simulink model "uz_ssi_interface_2025b"  (R2025b)
settings: Solver=FixedStepDiscrete  StartTime=0.0  StopTime=0.005  RelTol=1e-3
values from neighbouring files (symbols this model uses):
  f_ADC = 50e3    (= 50000)    [uz_ssi_interface_init.m]
  f_clock = 100e6    (= 100000000)    [uz_ssi_interface_init.m]
  t_ADC = 1/f_ADC    (= 2e-05)    [uz_ssi_interface_init.m]
  t_clock = 1/f_clock    (= 1e-08)    [uz_ssi_interface_init.m]
undefined symbols (not defined in the file or in its folder): binary_or_gray, bit_sum, delay_first_clk_on_off, PLL, ssi_clk_divider, ssi_encoder_bit_width_multi_turn, ssi_encoder_bit_width_single_turn, ssi_encoder_number_of_status_bits
libraries: hdlsllib x92, simulink x32, simulink_extras x7, spsSampleandHoldLib x1
(part 1 of 2)
settings Model: DataTypeOverride=Off  Creator=micha  LastModifiedBy=micha
settings SolverCC: AlgebraicLoopSolver=TrustRegion
settings DataIOCC: LimitDataPoints=on  SaveOutput=off  SaveTime=off
settings OptimizationCC: BlockReduction=off  ConditionallyExecuteInputs=off  DefaultParameterBehavior=Inlined  InheritOutputTypeSmallerThanSingle=on  LifeSpan=inf
settings DebuggingCC: AlgebraicLoopMsg=error  SingleTaskRateTransMsg=error  UnconnectedInputMsg=warning  UnconnectedOutputMsg=warning  UnconnectedLineMsg=warning  AllowSymbolicDim=off  StrictBusMsg=ErrorOnBusTreatedAsVector  SFUnexpectedBacktrackingDiag=warning  SFNoUnconditionalDefaultTransitionDiag=warning  SFExecutionAtInitializationDiag=none  ArithmeticOperatorsInVariantConditions=warning
settings HardwareCC: ProdBitPerPointer=32.0  ProdBitPerSizeT=32.0  ProdBitPerPtrDiffT=32.0  ProdLargestAtomicFloat=None  ProdIntDivRoundTo=Undefined  ProdEndianess=Unspecified  ProdWordSize=32.0  ProdHWDeviceType=ASIC/FPGA->ASIC/FPGA  ProdEqTarget=off
settings ModelReferenceCC: EnableRefExpFcnMdlSchedulingChecks=on
settings SFSimCC: SimUseLocalCustomCode=off  CustomCodeUndefinedFunction=UseInterfaceOnly
settings RTWCC: RTWUseLocalCustomCode=off  GPUComputeCapability=3.5  DLArmComputeVersion=19.05
settings CodeAppCC: StateflowObjectComments=on
settings GRTTargetCC: TargetLangStandard=C89/C90 (ANSI)
settings ConfigComp: CovScope=ReferencedModels  CovMetricSettings=dw  CovSaveCumulativeToWorkspaceVar=on  CovSaveSingleToWorkspaceVar=on  CovExternalEMLEnable=off  CovSFcnEnable=off

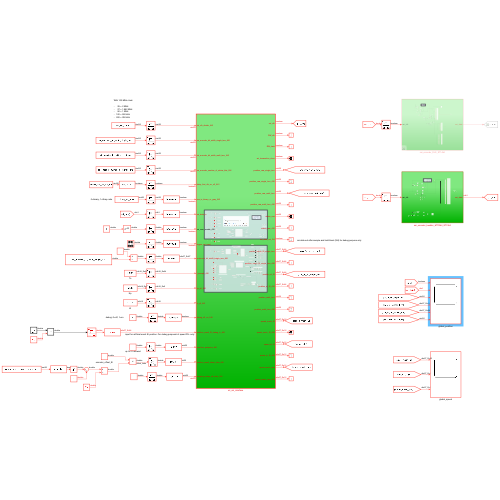
[thumbnail: Simulink's stored preview of the top-level diagram]
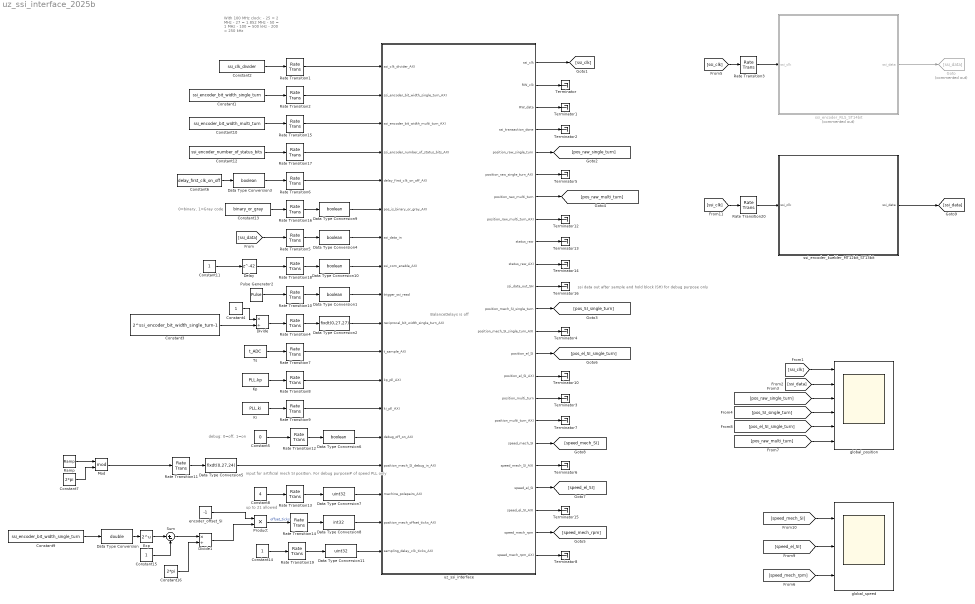
== system uz_ssi_interface_2025b ==
  note: input for artificial mech SI position. For debug purpose# of speed PLL only
  note: ssi data out after sample and hold block (SH) for debug purpose only
  note: up to 21 allowed
  note: debug: 0=off, 1=on
  note: BalanceDelays is off
  note: With 100 MHz clock:
      |
      | -     25 = 2 MHz
      | -     27 = 1.852 MHz
      | -     50 = 1 MHz
      | -   100 = 500 kHz
      | -   200 = 250 kHz
  note: 0=binary, 1=Gray code
  Constant1 : Constant  Value=ssi_encoder_bit_width_single_turn  OutDataTypeStr=uint32  SampleTime=t_clock
  Constant10 : Constant  Value=ssi_encoder_bit_width_multi_turn  OutDataTypeStr=uint32  SampleTime=t_clock
  Constant{4,11,14..15} (4 alike) : Constant  SampleTime=t_clock
  Constant12 : Constant  Value=ssi_encoder_number_of_status_bits  OutDataTypeStr=uint32  SampleTime=t_clock
  Constant13 : Constant  Value=binary_or_gray  OutDataTypeStr=uint32  SampleTime=t_clock
  Constant16 : Constant  Value=2*pi  SampleTime=t_clock
  Constant2 : Constant  Value=ssi_clk_divider  OutDataTypeStr=uint32  SampleTime=t_clock
  Constant3 : Constant  Value=2^ssi_encoder_bit_width_single_turn-1  OutDataTypeStr=double  SampleTime=t_clock
  Constant5 : Constant  Value=0  SampleTime=t_clock
  Constant6 : Constant  Value=delay_first_clk_on_off  OutDataTypeStr=uint32  SampleTime=t_clock
  Constant7 : Constant  Value=2*pi  SampleTime=t_clock
  Constant8 : Constant  Value=4  SampleTime=t_clock
  Constant9 : Constant  Value=ssi_encoder_bit_width_single_turn  OutDataTypeStr=uint32  SampleTime=t_clock
  Data Type Conversion : DataTypeConversion  OutDataTypeStr=double  SaturateOnIntegerOverflow=off  RndMeth=Floor
  Data Type Conversion{1,3..4,6,9..10} (6 alike) : DataTypeConversion  OutDataTypeStr=boolean  SaturateOnIntegerOverflow=off  RndMeth=Floor
  Data Type Conversion11 : DataTypeConversion  OutDataTypeStr=uint32  SaturateOnIntegerOverflow=off  RndMeth=Floor
  Data Type Conversion2 : DataTypeConversion  OutDataTypeStr=fixdt(0,27,27)  SaturateOnIntegerOverflow=off  RndMeth=Floor
  Data Type Conversion5 : DataTypeConversion  OutDataTypeStr=fixdt(0,27,24)  SaturateOnIntegerOverflow=off  RndMeth=Floor
  Data Type Conversion7 : DataTypeConversion  OutDataTypeStr=uint32  SaturateOnIntegerOverflow=off  RndMeth=Floor
  Data Type Conversion8 : DataTypeConversion  OutDataTypeStr=int32  SaturateOnIntegerOverflow=off  RndMeth=Floor
  Delay : Delay  DelayLength=42
  Divide : Product  Inputs=*/
  Divide1 : Product  Inputs=*/
  Exp : Math  Operator=2^u
  Goto : Goto  Commented=on  GotoTag=ssi_data
  Ki : Constant  Value=PLL.ki  OutDataTypeStr=fixdt(0,18,0)  SampleTime=-1
  Kp : Constant  Value=PLL.kp  OutDataTypeStr=fixdt(0,18,5)  SampleTime=-1
  Mod : Math  Operator=mod
  Product : Product
  Pulse Generator2 : DiscretePulseGenerator  Period=f_clock/f_ADC  PulseWidth=0.04*f_clock/f_ADC  PhaseDelay=250  SampleTime=t_clock
  Ramp : simulink/Sources/Ramp  slope=2*pi*100  start=7.5e-5  InitialOutput=0
  Rate Transition{1..20} (20 alike) : RateTransition  OutPortSampleTime=t_clock
  Sum : Sum  Inputs=|+-
  Terminator{,1..8,10,12..16} (15 alike) : Terminator
  Ts : Constant  Value=t_ADC  OutDataTypeStr=fixdt(0,18,24)  SampleTime=-1
  encoder_offset_SI : Constant  Value=-1  SampleTime=t_clock
  global_position : Scope  NumInputPorts=6
      settings: ActiveDisplayYMinimum=-0.125  ActiveDisplayYMaximum=1.125  DataLoggingVariableName=ScopeData2
  global_speed : Scope  NumInputPorts=3
      settings: ActiveDisplayYMinimum=-40.08166  ActiveDisplayYMaximum=351.59007
  ssi_encoder_RLS_ST14bit : Subsystem  Commented=on
  ssi_encoder_kuebler_MT12bit_ST13bit : Subsystem
  uz_ssi_interface : Subsystem  TreatAsAtomicUnit=on
  wires:
  Rate Transition10/1 -> Data Type Conversion1/1
  Pulse Generator2/1 -> Rate Transition10/1
  Constant2/1 -> Rate Transition1/1
  Rate Transition1/1 -> uz_ssi_interface/1(ssi_clk_divider_AXI)
  Constant1/1 -> Rate Transition2/1
  Rate Transition2/1 -> uz_ssi_interface/2(ssi_encoder_bit_width_single_turn_AXI)
  Rate Transition3/1 -> ssi_encoder_RLS_ST14bit/1(ssi_clk)
  ssi_encoder_RLS_ST14bit/1(ssi_data) -> Goto/1
  [ssi_data] -> Rate Transition5/1
  uz_ssi_interface/1(ssi_clk) -> [ssi_clk]
  uz_ssi_interface/3(RW_data) -> Terminator1/1
  uz_ssi_interface/4(ssi_transaction_done) -> Terminator2/1
  uz_ssi_interface/2(RW_clk) -> Terminator/1
  Data Type Conversion1/1 -> uz_ssi_interface/9(trigger_ssi_read)
  Rate Transition6/1 -> uz_ssi_interface/5(delay_first_clk_on_off_AXI)
  Data Type Conversion3/1 -> Rate Transition6/1
  Constant6/1 -> Data Type Conversion3/1
  uz_ssi_interface/6(position_raw_single_turn_AXI) -> Terminator5/1
  Rate Transition5/1 -> Data Type Conversion4/1
  Data Type Conversion4/1 -> uz_ssi_interface/7(ssi_data_in)
  Constant3/1 -> Divide/2
  Rate Transition4/1 -> Data Type Conversion2/1
  Data Type Conversion2/1 -> uz_ssi_interface/10(reciprocal_bit_width_single_turn_AXI)
  Constant4/1 -> Divide/1
  Divide/1 -> Rate Transition4/1
  uz_ssi_interface/13(position_mech_SI_single_turn_AXI) -> Terminator4/1
  Ts/1 -> Rate Transition7/1
  Rate Transition7/1 -> uz_ssi_interface/11(t_sample_AXI)
  Kp/1 -> Rate Transition8/1
  Rate Transition8/1 -> uz_ssi_interface/12(kp_pll_AXI)
  Ki/1 -> Rate Transition9/1
  Rate Transition9/1 -> uz_ssi_interface/13(ki_pll_AXI)
  uz_ssi_interface/18(speed_mech_SI) -> [speed_mech_SI]
  uz_ssi_interface/19(speed_mech_SI_AXI) -> Terminator6/1
  Rate Transition11/1 -> Data Type Conversion5/1
  Data Type Conversion5/1 -> uz_ssi_interface/15(position_mech_SI_debug_in_AXI)
  Data Type Conversion6/1 -> uz_ssi_interface/14(debug_off_on_AXI)
  Rate Transition12/1 -> Data Type Conversion6/1
  Constant5/1 -> Rate Transition12/1
  Mod/1 -> Rate Transition11/1
  Ramp/1 -> Mod/1
  Constant7/1 -> Mod/2
  uz_ssi_interface/23(speed_mech_rpm_AXI) -> Terminator8/1
  Rate Transition13/1 -> Data Type Conversion7/1
  Data Type Conversion7/1 -> uz_ssi_interface/16(machine_polepairs_AXI)
  Constant8/1 -> Rate Transition13/1
  Rate Transition14/1 -> Data Type Conversion8/1
  encoder_offset_SI/1 -> Product/1
  Data Type Conversion8/1 -> uz_ssi_interface/17(position_mech_offset_ticks_AXI)
  uz_ssi_interface/14(position_el_SI) -> [pos_el_SI_single_turn]
  uz_ssi_interface/15(position_el_SI_AXI) -> Terminator10/1
  Rate Transition15/1 -> uz_ssi_interface/3(ssi_encoder_bit_width_multi_turn_AXI)
  Constant10/1 -> Rate Transition15/1
  Rate Transition16/1 -> Data Type Conversion9/1
  Constant13/1 -> Rate Transition16/1
  Data Type Conversion9/1 -> uz_ssi_interface/6(pos_is_binary_or_gray_AXI)
  Rate Transition17/1 -> uz_ssi_interface/4(ssi_encoder_number_of_status_bits_AXI)
  Constant12/1 -> Rate Transition17/1
  Data Type Conversion10/1 -> uz_ssi_interface/8(ssi_com_enable_AXI)
  Rate Transition18/1 -> Data Type Conversion10/1
  Constant11/1 -> Delay/1
  uz_ssi_interface/7(position_raw_multi_turn) -> [pos_raw_multi_turn]
  uz_ssi_interface/8(position_raw_multi_turn_AXI) -> Terminator12/1
  uz_ssi_interface/9(status_raw) -> Terminator13/1
  uz_ssi_interface/10(status_raw_AXI) -> Terminator14/1
  uz_ssi_interface/21(speed_el_SI_AXI) -> Terminator15/1
  uz_ssi_interface/20(speed_el_SI) -> [speed_el_SI]
  [ssi_clk] -> global_position/1
  [ssi_data] -> global_position/2
  uz_ssi_interface/5(position_raw_single_turn) -> [pos_raw_single_turn]
  [pos_raw_single_turn] -> global_position/3
  [pos_SI_single_turn] -> global_position/4
  uz_ssi_interface/12(position_mech_SI_single_turn) -> [pos_SI_single_turn]
  uz_ssi_interface/11(ssi_data_out_SH) -> Terminator16/1
  uz_ssi_interface/22(speed_mech_rpm) -> [speed_mech_rpm]
  Delay/1 -> Rate Transition18/1
  [ssi_clk] -> Rate Transition3/1
  [speed_mech_rpm] -> global_speed/3
  [pos_raw_multi_turn] -> global_position/6
  [pos_el_SI_single_turn] -> global_position/5
  [speed_mech_SI] -> global_speed/1
  [speed_el_SI] -> global_speed/2
  Data Type Conversion11/1 -> uz_ssi_interface/18(sampling_delay_clk_ticks_AXI)
  Rate Transition19/1 -> Data Type Conversion11/1
  Constant14/1 -> Rate Transition19/1
  [ssi_clk] -> Rate Transition20/1
  Rate Transition20/1 -> ssi_encoder_kuebler_MT12bit_ST13bit/1(ssi_clk)
  ssi_encoder_kuebler_MT12bit_ST13bit/1(ssi_data) -> [ssi_data]
  uz_ssi_interface/16(position_multi_turn) -> Terminator3/1
  uz_ssi_interface/17(position_multi_turn_AXI) -> Terminator7/1
  Product/1 -> Rate Transition14/1  "offset_ticks"
  Constant9/1 -> Data Type Conversion/1
  Constant15/1 -> Sum/2
  Exp/1 -> Sum/1
  Sum/1 -> Divide1/1
  Constant16/1 -> Divide1/2
  Divide1/1 -> Product/2
  Data Type Conversion/1 -> Exp/1

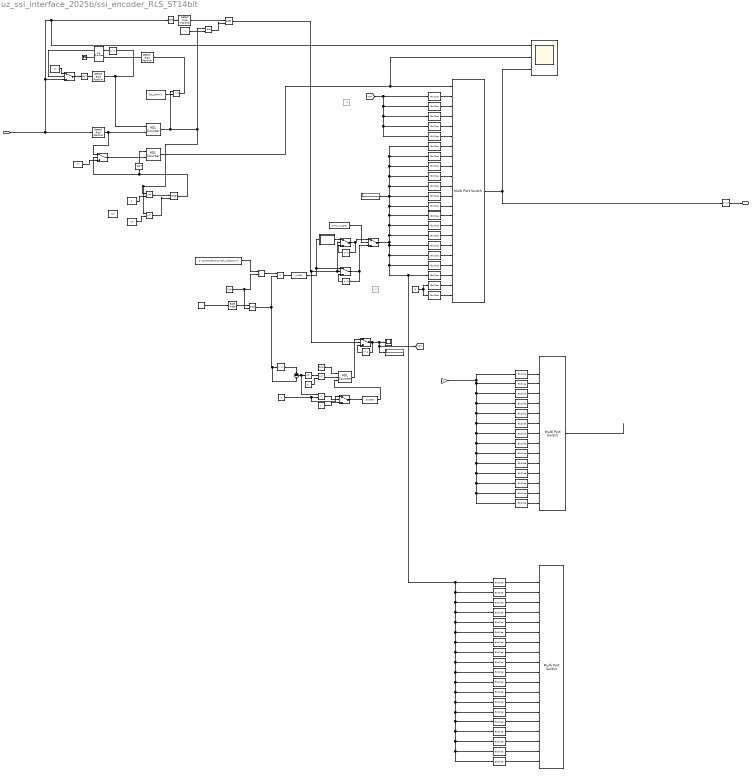
== system uz_ssi_interface_2025b/ssi_encoder_RLS_ST14bit ==
  note: 5bit multiturn, 14bit single turn 2bit status
  note: 14 bit single turn
  note: multiturn information
  note: 170 ns delay of the readhead
  note: Detect first falling edge of the clock
  note: singleturn information
  note: 19 bit single turn
  ssi_clk : Inport
  AND : Logic  IconShape=distinctive  AllPortsSameDT=off  OutDataTypeStr=boolean
  AND1 : Logic  IconShape=distinctive  AllPortsSameDT=off  OutDataTypeStr=boolean
  Abs : Abs  SaturateOnIntegerOverflow=off
  Bit Slice{1,14,19,26,40} (5 alike) : hdlsllib/Logic and Bit Operations/Bit Slice  lidx=1  ridx=1
  Bit Slice10 : hdlsllib/Logic and Bit Operations/Bit Slice  lidx=5  ridx=5
  Bit Slice{11,16,23,37} (4 alike) : hdlsllib/Logic and Bit Operations/Bit Slice  lidx=4  ridx=4
  Bit Slice{12,17,24,38} (4 alike) : hdlsllib/Logic and Bit Operations/Bit Slice  lidx=3  ridx=3
  Bit Slice{13,18,25,39} (4 alike) : hdlsllib/Logic and Bit Operations/Bit Slice  lidx=2  ridx=2
  Bit Slice{15,20..21,27,41} (5 alike) : hdlsllib/Logic and Bit Operations/Bit Slice  lidx=0  ridx=0
  Bit Slice2 : hdlsllib/Logic and Bit Operations/Bit Slice  lidx=13  ridx=13
  Bit Slice22 : hdlsllib/Logic and Bit Operations/Bit Slice  lidx=5  ridx=5
  Bit Slice28 : hdlsllib/Logic and Bit Operations/Bit Slice  lidx=13  ridx=13
  Bit Slice29 : hdlsllib/Logic and Bit Operations/Bit Slice  lidx=12  ridx=12
  Bit Slice3 : hdlsllib/Logic and Bit Operations/Bit Slice  lidx=12  ridx=12
  Bit Slice30 : hdlsllib/Logic and Bit Operations/Bit Slice  lidx=11  ridx=11
  Bit Slice31 : hdlsllib/Logic and Bit Operations/Bit Slice  lidx=10  ridx=10
  Bit Slice32 : hdlsllib/Logic and Bit Operations/Bit Slice  lidx=9  ridx=9
  Bit Slice33 : hdlsllib/Logic and Bit Operations/Bit Slice  lidx=8  ridx=8
  Bit Slice34 : hdlsllib/Logic and Bit Operations/Bit Slice  lidx=7  ridx=7
  Bit Slice35 : hdlsllib/Logic and Bit Operations/Bit Slice  lidx=6  ridx=6
  Bit Slice36 : hdlsllib/Logic and Bit Operations/Bit Slice  lidx=5  ridx=5
  Bit Slice4 : hdlsllib/Logic and Bit Operations/Bit Slice  lidx=11  ridx=11
  Bit Slice42 : hdlsllib/Logic and Bit Operations/Bit Slice  lidx=13  ridx=13
  Bit Slice43 : hdlsllib/Logic and Bit Operations/Bit Slice  lidx=12  ridx=12
  Bit Slice44 : hdlsllib/Logic and Bit Operations/Bit Slice  lidx=11  ridx=11
  Bit Slice45 : hdlsllib/Logic and Bit Operations/Bit Slice  lidx=10  ridx=10
  Bit Slice46 : hdlsllib/Logic and Bit Operations/Bit Slice  lidx=9  ridx=9
  Bit Slice47 : hdlsllib/Logic and Bit Operations/Bit Slice  lidx=8  ridx=8
  Bit Slice48 : hdlsllib/Logic and Bit Operations/Bit Slice  lidx=7  ridx=7
  Bit Slice49 : hdlsllib/Logic and Bit Operations/Bit Slice  lidx=6  ridx=6
  Bit Slice5 : hdlsllib/Logic and Bit Operations/Bit Slice  lidx=10  ridx=10
  Bit Slice50 : hdlsllib/Logic and Bit Operations/Bit Slice  lidx=18  ridx=18
  Bit Slice51 : hdlsllib/Logic and Bit Operations/Bit Slice  lidx=17  ridx=17
  Bit Slice52 : hdlsllib/Logic and Bit Operations/Bit Slice  lidx=16  ridx=16
  Bit Slice53 : hdlsllib/Logic and Bit Operations/Bit Slice  lidx=15  ridx=15
  Bit Slice54 : hdlsllib/Logic and Bit Operations/Bit Slice  lidx=14  ridx=14
  Bit Slice6 : hdlsllib/Logic and Bit Operations/Bit Slice  lidx=9  ridx=9
  Bit Slice7 : hdlsllib/Logic and Bit Operations/Bit Slice  lidx=8  ridx=8
  Bit Slice8 : hdlsllib/Logic and Bit Operations/Bit Slice  lidx=7  ridx=7
  Bit Slice9 : hdlsllib/Logic and Bit Operations/Bit Slice  lidx=6  ridx=6
  Constant : Constant  Value=bit_sum+1  SampleTime=t_clock
  Constant1 : Constant  Value=0  SampleTime=t_clock
  Constant10 : Constant  Value=false  SampleTime=t_clock
  Constant11 : Constant  Value=0  SampleTime=t_clock
  Constant12 : Constant  SampleTime=t_clock
  Constant13 : Constant  Value=0  OutDataTypeStr=uint32  SampleTime=t_clock
  Constant14 : Constant  Commented=on  Value=19  OutDataTypeStr=uint32  SampleTime=t_clock
  Constant15 : Constant  Value=binary_or_gray  SampleTime=t_clock
  Constant16 : Constant  Value=15  SampleTime=t_clock
  Constant2 : Constant  SampleTime=t_clock
  Constant3 : Constant  Value=0  OutDataTypeStr=boolean  SampleTime=t_clock
  Constant4 : Constant  Value=5  SampleTime=t_clock
  Constant5 : Constant  Value=2  SampleTime=t_clock
  Constant6 : Constant  Commented=on  Value=3875  OutDataTypeStr=uint32  SampleTime=t_clock
  Constant7 : Constant  Value=2*pi  SampleTime=t_clock
  Constant8 : Constant  Value=22  SampleTime=t_clock
  Constant9 : Constant  Value=2^ssi_encoder_bit_width_single_turn-1  SampleTime=t_clock
  Data Type Conversion : DataTypeConversion  OutDataTypeStr=uint32  SaturateOnIntegerOverflow=off  RndMeth=Floor
  Data Type Conversion1 : DataTypeConversion  OutDataTypeStr=boolean  SaturateOnIntegerOverflow=off  RndMeth=Floor
  Delay : Delay  DelayLength=1
  Delay1 : Delay  DelayLength=17  SampleTime=t_clock
  Delay2 : Delay  DelayLength=1  SampleTime=t_clock
  Delay3 : Delay  DelayLength=1
  Delay4 : Delay  DelayLength=1  InitialCondition=19  SampleTime=t_clock
  Delay5 : Delay  DelayLength=1  SampleTime=t_clock
  Detect Rise Positive{,1..3} (4 alike) : simulink/Logic and Bit Operations/Detect Rise Positive  vinit=0  OutDataTypeStr=boolean
  Display : Display
  Display1 : Display
  Divide : Product  Inputs=*/
  Gain : Gain
  HDL Counter : hdlsllib/Sources/HDL Counter  CountType=Count limited  CountInit=0  CountStep=1  CountMax=bit_sum+1  CountFromType=Initial value  CountFrom=0  CountResetPort=on  CountLoadPort=off  CountEnbPort=on  CountDirPort=off  CountHitOutputPort=off  CountDataType=Unsigned  CountWordLen=8  CountFracLen=0  CountSampTime=t_clock
  HDL Counter1 : hdlsllib/Sources/HDL Counter  CountType=Count limited  CountInit=0  CountStep=1  CountMax=bit_sum+1  CountFromType=Initial value  CountFrom=0  CountResetPort=on  CountLoadPort=off  CountEnbPort=on  CountDirPort=off  CountHitOutputPort=off  CountDataType=Unsigned  CountWordLen=8  CountFracLen=0  CountSampTime=t_clock
  HDL Counter2 : hdlsllib/Sources/HDL Counter  CountType=Count limited  CountInit=19  CountStep=1  CountMax=ssi_encoder_bit_width_multi_turn  CountFromType=Initial value  CountFrom=19  CountResetPort=on  CountLoadPort=off  CountEnbPort=on  CountDirPort=on  CountHitOutputPort=off  CountDataType=Unsigned  CountWordLen=5  CountFracLen=0  CountSampTime=t_clock
  Index Vector : MultiPortSwitch  DataPortOrder=Zero-based contiguous  Inputs=21  zeroidx=on  SaturateOnIntegerOverflow=off  InputSameDT=off
  Index Vector1 : MultiPortSwitch  DataPortOrder=Zero-based contiguous  Inputs=14  zeroidx=on  SaturateOnIntegerOverflow=off  InputSameDT=off
  Index Vector2 : MultiPortSwitch  DataPortOrder=Zero-based contiguous  Inputs=19  zeroidx=on  SaturateOnIntegerOverflow=off  InputSameDT=off
  MATLAB Function : MATLAB Function  TreatAsAtomicUnit=on
  Mod : Math  Operator=mod
  NOT : Logic  Operator=NOT  IconShape=distinctive  AllPortsSameDT=off  OutDataTypeStr=boolean
  NOT1 : Logic  Operator=NOT  IconShape=distinctive  AllPortsSameDT=off  OutDataTypeStr=boolean
  NOT2 : Logic  Operator=NOT  IconShape=distinctive  AllPortsSameDT=off  OutDataTypeStr=boolean
  Product : Product
  Ramp : simulink/Sources/Ramp  slope=-2*pi*50  start=7.5e-5  InitialOutput=0
  Rate Transition : RateTransition  OutPortSampleTime=t_clock
  Relational Operator : RelationalOperator  OutDataTypeStr=boolean  RndMeth=Simplest  InputSameDT=off
  Relational Operator1 : RelationalOperator  OutDataTypeStr=boolean  RndMeth=Simplest  InputSameDT=off
  Relational Operator2 : RelationalOperator  Operator===  OutDataTypeStr=boolean  RndMeth=Simplest  InputSameDT=off
  Relational Operator3 : RelationalOperator  Operator=<=  OutDataTypeStr=boolean  RndMeth=Simplest  InputSameDT=off
  Relational Operator4 : RelationalOperator  OutDataTypeStr=boolean  RndMeth=Simplest  InputSameDT=off
  Relational Operator5 : RelationalOperator  Operator=<  OutDataTypeStr=boolean  RndMeth=Simplest  InputSameDT=off
  S-R Flip-Flop : simulink_extras/Flip Flops/S-R Flip-Flop  initial_condition=0
  Scope : Scope  NumInputPorts=3
      settings: ActiveDisplayYMinimum=-2.5  ActiveDisplayYMaximum=22.5
  Scope1 : Scope
  Sum : Sum  Inputs=+-
  Switch{,1..6} (7 alike) : Switch  Criteria=u2 > Threshold  SaturateOnIntegerOverflow=off  InputSameDT=off
  Terminator : Terminator
  ssi_data : Outport
  wires:
  NOT/1 -> Detect Rise Positive/1
  Constant/1 -> Relational Operator/2
  Switch/1 -> NOT/1
  S-R Flip-Flop/1 -> Switch/2
  Delay/1 -> S-R Flip-Flop/1
  Relational Operator/1 -> Detect Rise Positive2/1
  Detect Rise Positive2/1 -> S-R Flip-Flop/2
  Detect Rise Positive/1 -> HDL Counter/1, Delay/1
  Relational Operator2/1 -> AND/2
  Constant2/1 -> Relational Operator2/2
  NOT1/1 -> Detect Rise Positive3/1
  Detect Rise Positive3/1 -> AND/1
  Detect Rise Positive1/1 -> HDL Counter/2, Switch3/1
  HDL Counter/1 -> Relational Operator3/1, Relational Operator1/1, Relational Operator2/1, Relational Operator/1
  S-R Flip-Flop/2 -> Terminator/1
  Constant1/1 -> Switch/1
  ssi_clk/1 -> Scope/1, NOT1/1, Switch/3, Detect Rise Positive1/1
  Relational Operator1/1 -> AND1/1
  AND1/1 -> NOT2/1, Switch3/2
  Constant5/1 -> Relational Operator1/2
  Relational Operator3/1 -> AND1/2
  Constant16/1 -> Relational Operator3/2
  Switch3/1 -> HDL Counter1/2
  NOT2/1 -> HDL Counter1/1
  Ramp/1 -> Rate Transition/1
  Constant9/1 -> Divide/1
  Divide/1 -> Product/1
  Constant7/1 -> Mod/2, Divide/2
  Product/1 -> Data Type Conversion/1
  Rate Transition/1 -> Mod/1
  Delay2/1 -> Switch1/3
  Data Type Conversion/1 -> Switch1/1, MATLAB Function/1(u)
  AND/1 -> Switch2/2, Switch6/2, Switch1/2
  Constant3/1 -> Switch3/3
  HDL Counter1/1 -> Scope/2, Index Vector/1
  Delay1/1 -> ssi_data/1
  Delay3/1 -> Sum/1
  Mod/1 -> Sum/2, Delay3/1, Product/2
  Sum/1 -> Relational Operator5/1, Abs/1
  Abs/1 -> Relational Operator4/1
  Constant4/1 -> Relational Operator4/2
  Relational Operator4/1 -> HDL Counter2/2
  HDL Counter2/1 -> Switch2/1
  Delay4/1 -> Switch2/3
  Switch2/1 -> [MT], Display1/1, Scope1/1, Delay4/1
  Constant10/1 -> HDL Counter2/1
  Constant11/1 -> Switch4/1, Relational Operator5/2
  Relational Operator5/1 -> Switch4/2
  Switch4/1 -> Data Type Conversion1/1
  Constant12/1 -> Switch4/3
  [MT] -> Bit Slice17/1, Bit Slice18/1, Bit Slice19/1, Bit Slice20/1, Bit Slice16/1
  Bit Slice16/1 -> Index Vector/2
  Bit Slice17/1 -> Index Vector/3
  Bit Slice18/1 -> Index Vector/4
  Bit Slice19/1 -> Index Vector/5
  Bit Slice20/1 -> Index Vector/6
  Bit Slice2/1 -> Index Vector/7
  Bit Slice3/1 -> Index Vector/8
  Bit Slice4/1 -> Index Vector/9
  Bit Slice5/1 -> Index Vector/10
  Bit Slice6/1 -> Index Vector/11
  Bit Slice7/1 -> Index Vector/12
  Bit Slice8/1 -> Index Vector/13
  Bit Slice9/1 -> Index Vector/14
  Bit Slice10/1 -> Index Vector/15
  Bit Slice11/1 -> Index Vector/16
  Bit Slice12/1 -> Index Vector/17
  Bit Slice13/1 -> Index Vector/18
  Bit Slice14/1 -> Index Vector/19
  Bit Slice15/1 -> Index Vector/20
  Bit Slice1/1 -> Index Vector/21
  Bit Slice21/1 -> Index Vector/22
  Constant13/1 -> Bit Slice1/1, Bit Slice21/1
  Data Type Conversion1/1 -> HDL Counter2/3
  Constant15/1 -> Switch5/2
  Switch1/1 -> Delay2/1, Switch5/3
  MATLAB Function/1(y) -> Switch6/1
  Switch6/1 -> Delay5/1, Switch5/1
  Delay5/1 -> Switch6/3
  Bit Slice29/1 -> Index Vector1/3
  Bit Slice33/1 -> Index Vector1/7
  Bit Slice26/1 -> Index Vector1/14
  Bit Slice22/1 -> Index Vector1/10
  Bit Slice28/1 -> Index Vector1/2
  Bit Slice34/1 -> Index Vector1/8
  Bit Slice23/1 -> Index Vector1/11
  Bit Slice31/1 -> Index Vector1/5
  Bit Slice27/1 -> Index Vector1/15
  Bit Slice35/1 -> Index Vector1/9
  Bit Slice30/1 -> Index Vector1/4
  Bit Slice32/1 -> Index Vector1/6
  Bit Slice25/1 -> Index Vector1/13
  Bit Slice24/1 -> Index Vector1/12
  Index Vector1/1 -> ?
  Bit Slice47/1 -> Index Vector2/12
  Bit Slice37/1 -> Index Vector2/16
  Bit Slice40/1 -> Index Vector2/19
  Bit Slice36/1 -> Index Vector2/15
  Bit Slice44/1 -> Index Vector2/9
  Bit Slice41/1 -> Index Vector2/20
  Bit Slice42/1 -> Index Vector2/7
  Bit Slice38/1 -> Index Vector2/17
  Bit Slice45/1 -> Index Vector2/10
  Bit Slice46/1 -> Index Vector2/11
  Bit Slice48/1 -> Index Vector2/13
  Bit Slice43/1 -> Index Vector2/8
  Bit Slice49/1 -> Index Vector2/14
  Bit Slice39/1 -> Index Vector2/18
  Bit Slice52/1 -> Index Vector2/4
  Bit Slice53/1 -> Index Vector2/5
  Bit Slice50/1 -> Index Vector2/2
  Bit Slice54/1 -> Index Vector2/6
  Bit Slice51/1 -> Index Vector2/3
  Switch5/1 -> Bit Slice37/1, Bit Slice38/1, Bit Slice39/1, Bit Slice40/1, Bit Slice41/1, Bit Slice36/1, Bit Slice49/1, Bit Slice48/1, Bit Slice47/1, Bit Slice46/1, Bit Slice45/1, Bit Slice44/1, Bit Slice43/1, Bit Slice42/1, Bit Slice54/1, Bit Slice53/1, Bit Slice52/1, Bit Slice51/1, Bit Slice50/1, Bit Slice15/1, Bit Slice14/1, Bit Slice13/1, Bit Slice12/1, Display/1, Bit Slice6/1, Bit Slice5/1, Bit Slice4/1, Bit Slice2/1, Bit Slice3/1, Bit Slice7/1, Bit Slice8/1, Bit Slice9/1, Bit Slice10/1, Bit Slice11/1
  Index Vector/1 -> Scope/3, Delay1/1
  Gain/1 -> Bit Slice28/1, Bit Slice27/1, Bit Slice26/1, Bit Slice25/1, Bit Slice24/1, Bit Slice23/1, Bit Slice22/1, Bit Slice35/1, Bit Slice34/1, Bit Slice33/1, Bit Slice32/1, Bit Slice31/1, Bit Slice30/1, Bit Slice29/1

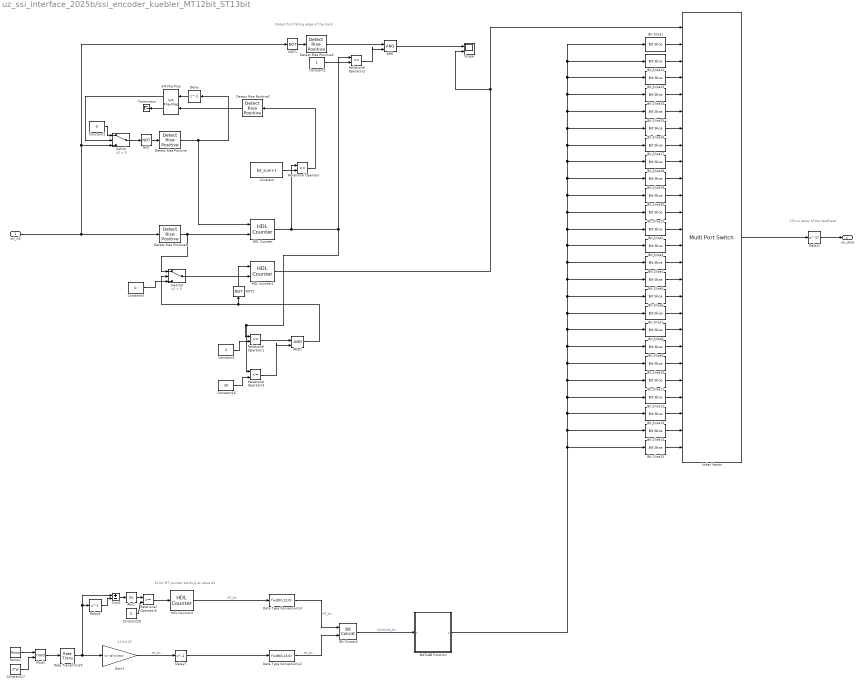
== system uz_ssi_interface_2025b/ssi_encoder_kuebler_MT12bit_ST13bit ==
  note: 12 bit MT counter starting at value 42
  note: 170 ns delay of the readhead
  note: Detect first falling edge of the clock
  note: 13 bit ST
  ssi_clk : Inport
  AND : Logic  IconShape=distinctive  AllPortsSameDT=off  OutDataTypeStr=boolean
  AND1 : Logic  IconShape=distinctive  AllPortsSameDT=off  OutDataTypeStr=boolean
  Abs1 : Abs  SaturateOnIntegerOverflow=off
  Bit Concat4 : hdlsllib/Logic and Bit Operations/Bit Concat  numInputs=2
  Bit Slice1 : hdlsllib/Logic and Bit Operations/Bit Slice  lidx=24  ridx=24
  Bit Slice10 : hdlsllib/Logic and Bit Operations/Bit Slice  lidx=5  ridx=5
  Bit Slice11 : hdlsllib/Logic and Bit Operations/Bit Slice  lidx=4  ridx=4
  Bit Slice12 : hdlsllib/Logic and Bit Operations/Bit Slice  lidx=3  ridx=3
  Bit Slice13 : hdlsllib/Logic and Bit Operations/Bit Slice  lidx=2  ridx=2
  Bit Slice14 : hdlsllib/Logic and Bit Operations/Bit Slice  lidx=1  ridx=1
  Bit Slice15 : hdlsllib/Logic and Bit Operations/Bit Slice  lidx=0  ridx=0
  Bit Slice2 : hdlsllib/Logic and Bit Operations/Bit Slice  lidx=13  ridx=13
  Bit Slice21 : hdlsllib/Logic and Bit Operations/Bit Slice  lidx=23  ridx=23
  Bit Slice22 : hdlsllib/Logic and Bit Operations/Bit Slice  lidx=14  ridx=14
  Bit Slice23 : hdlsllib/Logic and Bit Operations/Bit Slice  lidx=22  ridx=22
  Bit Slice24 : hdlsllib/Logic and Bit Operations/Bit Slice  lidx=21  ridx=21
  Bit Slice25 : hdlsllib/Logic and Bit Operations/Bit Slice  lidx=20  ridx=20
  Bit Slice26 : hdlsllib/Logic and Bit Operations/Bit Slice  lidx=19  ridx=19
  Bit Slice27 : hdlsllib/Logic and Bit Operations/Bit Slice  lidx=18  ridx=18
  Bit Slice28 : hdlsllib/Logic and Bit Operations/Bit Slice  lidx=17  ridx=17
  Bit Slice29 : hdlsllib/Logic and Bit Operations/Bit Slice  lidx=16  ridx=16
  Bit Slice3 : hdlsllib/Logic and Bit Operations/Bit Slice  lidx=12  ridx=12
  Bit Slice30 : hdlsllib/Logic and Bit Operations/Bit Slice  lidx=15  ridx=15
  Bit Slice4 : hdlsllib/Logic and Bit Operations/Bit Slice  lidx=11  ridx=11
  Bit Slice5 : hdlsllib/Logic and Bit Operations/Bit Slice  lidx=10  ridx=10
  Bit Slice6 : hdlsllib/Logic and Bit Operations/Bit Slice  lidx=9  ridx=9
  Bit Slice7 : hdlsllib/Logic and Bit Operations/Bit Slice  lidx=8  ridx=8
  Bit Slice8 : hdlsllib/Logic and Bit Operations/Bit Slice  lidx=7  ridx=7
  Bit Slice9 : hdlsllib/Logic and Bit Operations/Bit Slice  lidx=6  ridx=6
  Constant : Constant  Value=bit_sum+1  SampleTime=t_clock
  Constant1 : Constant  Value=0  SampleTime=t_clock
  Constant16 : Constant  Value=26  SampleTime=t_clock
  Constant17 : Constant  Value=2*pi  SampleTime=t_clock
  Constant18 : Constant  Value=5  SampleTime=t_clock
  Constant2 : Constant  SampleTime=t_clock
  Constant3 : Constant  Value=0  OutDataTypeStr=boolean  SampleTime=t_clock
  Constant5 : Constant  Value=2  SampleTime=t_clock
  Data Type Conversion12 : DataTypeConversion  OutDataTypeStr=fixdt(0,13,0)  SaturateOnIntegerOverflow=off  RndMeth=Floor
  Data Type Conversion13 : DataTypeConversion  OutDataTypeStr=fixdt(0,12,0)  SaturateOnIntegerOverflow=off  RndMeth=Floor
  Delay : Delay  DelayLength=1
  Delay1 : Delay  DelayLength=17  SampleTime=t_clock
  Delay6 : Delay  DelayLength=1
  Delay7 : Delay  DelayLength=1
  Detect Rise Positive{,1..3} (4 alike) : simulink/Logic and Bit Operations/Detect Rise Positive  vinit=0  OutDataTypeStr=boolean
  Gain1 : Gain  Gain=((2^13)-1)/(2*pi)  OutDataTypeStr=uint32
  HDL Counter : hdlsllib/Sources/HDL Counter  CountType=Count limited  CountInit=0  CountStep=1  CountMax=bit_sum+1  CountFromType=Initial value  CountFrom=0  CountResetPort=on  CountLoadPort=off  CountEnbPort=on  CountDirPort=off  CountHitOutputPort=off  CountDataType=Unsigned  CountWordLen=8  CountFracLen=0  CountSampTime=t_clock
  HDL Counter1 : hdlsllib/Sources/HDL Counter  CountType=Count limited  CountInit=0  CountStep=1  CountMax=bit_sum+1  CountFromType=Initial value  CountFrom=0  CountResetPort=on  CountLoadPort=off  CountEnbPort=on  CountDirPort=off  CountHitOutputPort=off  CountDataType=Unsigned  CountWordLen=8  CountFracLen=0  CountSampTime=t_clock
  HDL Counter3 : hdlsllib/Sources/HDL Counter  CountType=Count limited  CountInit=42  CountStep=1  CountMax=4095  CountFromType=Initial value  CountFrom=42  CountResetPort=off  CountLoadPort=off  CountEnbPort=on  CountDirPort=off  CountHitOutputPort=off  CountDataType=Unsigned  CountWordLen=12  CountFracLen=0  CountSampTime=1
  Index Vector : MultiPortSwitch  DataPortOrder=Zero-based contiguous  Inputs=25  zeroidx=on  SaturateOnIntegerOverflow=off  InputSameDT=off
  MATLAB Function : MATLAB Function  TreatAsAtomicUnit=on
  Mod1 : Math  Operator=mod
  NOT : Logic  Operator=NOT  IconShape=distinctive  AllPortsSameDT=off  OutDataTypeStr=boolean
  NOT1 : Logic  Operator=NOT  IconShape=distinctive  AllPortsSameDT=off  OutDataTypeStr=boolean
  NOT2 : Logic  Operator=NOT  IconShape=distinctive  AllPortsSameDT=off  OutDataTypeStr=boolean
  Ramp1 : simulink/Sources/Ramp  slope=2*pi*50  start=0  InitialOutput=0
  Rate Transition20 : RateTransition  OutPortSampleTime=t_clock
  Relational Operator : RelationalOperator  OutDataTypeStr=boolean  RndMeth=Simplest  InputSameDT=off
  Relational Operator1 : RelationalOperator  OutDataTypeStr=boolean  RndMeth=Simplest  InputSameDT=off
  Relational Operator2 : RelationalOperator  Operator===  OutDataTypeStr=boolean  RndMeth=Simplest  InputSameDT=off
  Relational Operator3 : RelationalOperator  Operator=<=  OutDataTypeStr=boolean  RndMeth=Simplest  InputSameDT=off
  Relational Operator6 : RelationalOperator  OutDataTypeStr=boolean  RndMeth=Simplest  InputSameDT=off
  S-R Flip-Flop : simulink_extras/Flip Flops/S-R Flip-Flop  initial_condition=0
  Scope : Scope  NumInputPorts=2
      settings: ActiveDisplayYMinimum=-0.125  ActiveDisplayYMaximum=1.125
  Sum1 : Sum  Inputs=+-
  Switch : Switch  Criteria=u2 > Threshold  SaturateOnIntegerOverflow=off  InputSameDT=off
  Switch3 : Switch  Criteria=u2 > Threshold  SaturateOnIntegerOverflow=off  InputSameDT=off
  Terminator : Terminator
  ssi_data : Outport
  wires:
  NOT/1 -> Detect Rise Positive/1
  Constant/1 -> Relational Operator/2
  Switch/1 -> NOT/1
  S-R Flip-Flop/1 -> Switch/2
  Delay/1 -> S-R Flip-Flop/1
  Relational Operator/1 -> Detect Rise Positive2/1
  Detect Rise Positive2/1 -> S-R Flip-Flop/2
  Detect Rise Positive/1 -> HDL Counter/1, Delay/1
  Relational Operator2/1 -> AND/2
  Constant2/1 -> Relational Operator2/2
  NOT1/1 -> Detect Rise Positive3/1
  Detect Rise Positive3/1 -> AND/1
  Detect Rise Positive1/1 -> HDL Counter/2, Switch3/1
  HDL Counter/1 -> Relational Operator3/1, Relational Operator1/1, Relational Operator2/1, Relational Operator/1
  S-R Flip-Flop/2 -> Terminator/1
  Constant1/1 -> Switch/1
  ssi_clk/1 -> NOT1/1, Switch/3, Detect Rise Positive1/1
  Relational Operator1/1 -> AND1/1
  AND1/1 -> NOT2/1, Switch3/2
  Constant5/1 -> Relational Operator1/2
  Relational Operator3/1 -> AND1/2
  Constant16/1 -> Relational Operator3/2
  Switch3/1 -> HDL Counter1/2
  NOT2/1 -> HDL Counter1/1
  Constant3/1 -> Switch3/3
  Delay1/1 -> ssi_data/1
  Constant17/1 -> Mod1/2
  Delay6/1 -> Sum1/2
  HDL Counter3/1 -> Data Type Conversion13/1  "MT_bin"
  Ramp1/1 -> Mod1/1
  Gain1/1 -> Delay7/1  "ST_bin"
  Data Type Conversion12/1 -> Bit Concat4/2  "ST_bin"
  Constant18/1 -> Relational Operator6/2
  Mod1/1 -> Rate Transition20/1
  Abs1/1 -> Relational Operator6/1
  Sum1/1 -> Abs1/1
  Delay7/1 -> Data Type Conversion12/1
  Rate Transition20/1 -> Sum1/1, Delay6/1, Gain1/1
  Data Type Conversion13/1 -> Bit Concat4/1  "MT_bin"
  Relational Operator6/1 -> HDL Counter3/1
  HDL Counter1/1 -> Index Vector/1, Scope/2
  Index Vector/1 -> Delay1/1
  AND/1 -> Scope/1
  Bit Slice6/1 -> Index Vector/17
  Bit Slice5/1 -> Index Vector/16
  Bit Slice2/1 -> Index Vector/13
  Bit Slice9/1 -> Index Vector/20
  Bit Slice3/1 -> Index Vector/14
  Bit Slice8/1 -> Index Vector/19
  Bit Slice24/1 -> Index Vector/5
  Bit Slice26/1 -> Index Vector/7
  Bit Slice23/1 -> Index Vector/4
  Bit Slice22/1 -> Index Vector/12
  Bit Slice15/1 -> Index Vector/26
  Bit Slice27/1 -> Index Vector/8
  Bit Slice14/1 -> Index Vector/25
  Bit Slice25/1 -> Index Vector/6
  Bit Slice28/1 -> Index Vector/9
  Bit Slice4/1 -> Index Vector/15
  Bit Slice10/1 -> Index Vector/21
  Bit Slice7/1 -> Index Vector/18
  Bit Slice30/1 -> Index Vector/11
  Bit Slice13/1 -> Index Vector/24
  Bit Slice29/1 -> Index Vector/10
  Bit Slice11/1 -> Index Vector/22
  Bit Slice12/1 -> Index Vector/23
  Bit Slice21/1 -> Index Vector/3
  Bit Slice1/1 -> Index Vector/2
  Bit Concat4/1 -> MATLAB Function/1(u)  "Combined_bin"
  MATLAB Function/1(y) -> Bit Slice15/1, Bit Slice14/1, Bit Slice13/1, Bit Slice11/1, Bit Slice10/1, Bit Slice8/1, Bit Slice7/1, Bit Slice6/1, Bit Slice5/1, Bit Slice4/1, Bit Slice3/1, Bit Slice2/1, Bit Slice22/1, Bit Slice30/1, Bit Slice29/1, Bit Slice28/1, Bit Slice27/1, Bit Slice26/1, Bit Slice25/1, Bit Slice24/1, Bit Slice23/1, Bit Slice21/1, Bit Slice1/1, Bit Slice9/1, Bit Slice12/1

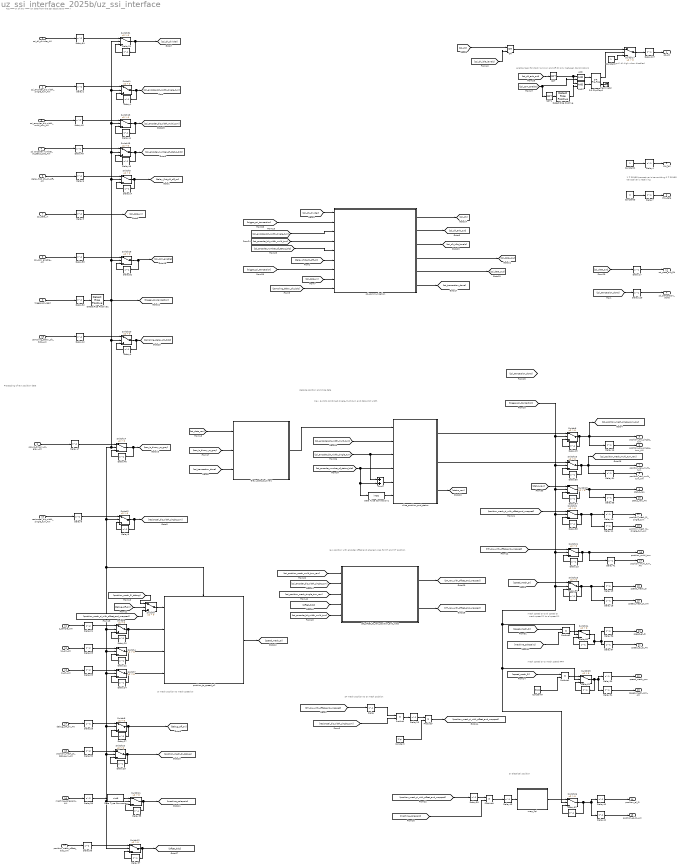
== system uz_ssi_interface_2025b/uz_ssi_interface ==
  note: enable logic for clock: turns on and off clk only between transmissions
  note: pull clk high when disabled
  note: ST mech position to SI mech position
  note: 1 = RS485 transceiver is transmitting
      | 0 = RS485 transceiver is receiving
  note: Acquisition of raw position data from the SSI absolute encoder
  note: SI mech position to mech speed SI
  note: mech speed SI to mech speed RPM
  note: SI electrical position
  note: mech speed SI to el speed SI
  note: max. 64 bits combined
      | single-/multi-turn and status bit width
  note: decode position and slice data
  note: mech speed SI to el speed SI
  note: Processing of raw position data
  note: raw position with encoder offset and aligned wrap for ST and MT position
  ssi_clk_divider_AXI : Inport  OutDataTypeStr=uint32
  ssi_encoder_bit_width_single_turn_AXI : Inport  Port=2  OutDataTypeStr=uint32
  ssi_encoder_bit_width_multi_turn_AXI : Inport  Port=3  OutDataTypeStr=uint32
  ssi_encoder_number_of_status_bits_AXI : Inport  Port=4  OutDataTypeStr=uint32
  delay_first_clk_on_off_AXI : Inport  Port=5  OutDataTypeStr=boolean
  pos_is_binary_or_gray_AXI : Inport  Port=6  OutDataTypeStr=boolean
  ssi_data_in : Inport  Port=7
  ssi_com_enable_AXI : Inport  Port=8  OutDataTypeStr=boolean
  trigger_ssi_read : Inport  Port=9  OutDataTypeStr=boolean
  reciprocal_bit_width_single_turn_AXI : Inport  Port=10
  t_sample_AXI : Inport  Port=11
  kp_pll_AXI : Inport  Port=12
  ki_pll_AXI : Inport  Port=13
  debug_off_on_AXI : Inport  Port=14
  position_mech_SI_debug_in_AXI : Inport  Port=15
  machine_polepairs_AXI : Inport  Port=16
  position_mech_offset_ticks_AXI : Inport  Port=17
  sampling_delay_clk_ticks_AXI : Inport  Port=18  OutDataTypeStr=uint32
  AND : Logic  IconShape=distinctive  AllPortsSameDT=off  OutDataTypeStr=boolean
  AND1 : Logic  IconShape=distinctive  AllPortsSameDT=off  OutDataTypeStr=boolean
  Constant : Constant  Value=2*pi  OutDataTypeStr=fixdt(0,18,15)  SampleTime=t_clock
  Constant1 : Constant  OutDataTypeStr=boolean  SampleTime=t_clock
  Constant3 : Constant  Value=0  OutDataTypeStr=boolean  SampleTime=t_clock
  Constant4 : Constant  Value=30/pi  OutDataTypeStr=fixdt(0,18,14)  SampleTime=-1
  Constant5 : Constant  OutDataTypeStr=boolean  SampleTime=t_clock
  Data Type Conversion : DataTypeConversion  OutDataTypeStr=uint8  SaturateOnIntegerOverflow=off  RndMeth=Floor
  Data Type Conversion1 : DataTypeConversion  OutDataTypeStr=int32  SaturateOnIntegerOverflow=off  RndMeth=Floor
  Delay{,20,22,24,26..27,29,37} (8 alike) : Delay  DelayLength=1  InitialCondition=0
  Delay1 : Delay  DelayLength=1  InitialCondition=ssi_encoder_bit_width_single_turn
  Delay{4,7..8,10..11,16..19,33..34,39..40,42..43,56..62,127,129} (24 alike) : Delay  DelayLength=1
  Delay12 : Delay  InitialCondition=uint32(0)
  Delay{5,13,15,41,50..51,54..55} (8 alike) : Delay  DelayLength=1  InitialCondition=uint32(0)
  Delay14 : Delay  DelayLength=1  InitialCondition=delay_first_clk_on_off
  Delay{2..3,6,9,21,23,25,28,30,32,36,38,45,47,53,64} (16 alike) : Delay
  Delay31 : Delay  DelayLength=1  InitialCondition=ssi_clk_divider
  Delay35 : Delay  DelayLength=1  InitialCondition=1
  Delay44 : Delay  DelayLength=1  InitialCondition=ssi_encoder_bit_width_multi_turn
  Delay46 : Delay  DelayLength=1  InitialCondition=false
  Delay48 : Delay  DelayLength=1  InitialCondition=uint32(ssi_encoder_number_of_status_bits)
  Delay49 : Delay  InitialCondition=uint32(0)
  Delay52 : Delay  DelayLength=1  InitialCondition=false
  Detect Rise Positive : simulink/Logic and Bit Operations/Detect Rise Positive  vinit=0  OutDataTypeStr=boolean
  Detect Rise Positive1 : simulink/Logic and Bit Operations/Detect Rise Positive  vinit=0  OutDataTypeStr=boolean
  Gray_code_to_binary : Subsystem
  NOT : Logic  Operator=NOT  IconShape=distinctive  AllPortsSameDT=off  OutDataTypeStr=boolean
  NOT1 : Logic  Operator=NOT  IconShape=distinctive  AllPortsSameDT=off  OutDataTypeStr=boolean
  OR : Logic  Operator=OR  IconShape=distinctive  AllPortsSameDT=off  OutDataTypeStr=boolean
  Product : Product  OutDataTypeStr=fixdt(0,27,24)
  Product1 : Product  OutDataTypeStr=fixdt(1,27,12)
  Product2 : Product  OutDataTypeStr=fixdt(1,27,12)
  Product4 : Product  OutDataTypeStr=fixdt(0,27,20)
  Product7 : Product  OutDataTypeStr=fixdt(0,27,24)
  S-R Flip-Flop1 : simulink_extras/Flip Flops/S-R Flip-Flop  initial_condition=0
  Sum2 : Sum  OutDataTypeStr=int32
  Switch{1..26,31} (27 alike) : Switch  Criteria=u2 > Threshold  SaturateOnIntegerOverflow=off  InputSameDT=off
  Terminator : Terminator
  position_to_speed_pll : Subsystem  TreatAsAtomicUnit=on
      settings: LibrarySourceBlock=|
      | hdlsllib/Ports &
      | Subsystems/Triggered
      | Subsystem
  set_offset_to_raw_position_and_wrap : Subsystem
  slice_position_and_status : Subsystem
      settings: LibrarySourceBlock=|
      | hdlsllib/Ports &
      | Subsystems/Subsystem
  ssi_communication : Subsystem
  wrap_2pi : Subsystem
  ssi_clk : Outport
  RW_clk : Outport  Port=2
  RW_data : Outport  Port=3
  ssi_transaction_done : Outport  Port=4  OutDataTypeStr=boolean  LockScale=on
  position_raw_single_turn : Outport  Port=5  OutDataTypeStr=uint32  LockScale=on
  position_raw_single_turn_AXI : Outport  Port=6  OutDataTypeStr=uint32  LockScale=on
  position_raw_multi_turn : Outport  Port=7  OutDataTypeStr=uint32  LockScale=on
  position_raw_multi_turn_AXI : Outport  Port=8  OutDataTypeStr=uint32  LockScale=on
  status_raw : Outport  Port=9  OutDataTypeStr=uint32  LockScale=on
  status_raw_AXI : Outport  Port=10  OutDataTypeStr=uint32  LockScale=on
  ssi_data_out_SH : Outport  Port=11
  position_mech_SI_single_turn : Outport  Port=12
  position_mech_SI_single_turn_AXI : Outport  Port=13
  position_el_SI : Outport  Port=14
  position_el_SI_AXI : Outport  Port=15
  position_multi_turn : Outport  Port=16  OutDataTypeStr=uint32  LockScale=on
  position_multi_turn_AXI : Outport  Port=17  OutDataTypeStr=uint32  LockScale=on
  speed_mech_SI : Outport  Port=18
  speed_mech_SI_AXI : Outport  Port=19
  speed_el_SI : Outport  Port=20
  speed_el_SI_AXI : Outport  Port=21
  speed_mech_rpm : Outport  Port=22
  speed_mech_rpm_AXI : Outport  Port=23
  wires:
  Delay129/1 -> ssi_transaction_done/1
  trigger_ssi_read/1 -> Delay32/1
  Delay32/1 -> Detect Rise Positive1/1
  Delay64/1 -> Switch31/1
  ssi_clk_divider_AXI/1 -> Delay64/1
  Delay31/1 -> Switch31/3
  Switch31/1 -> Delay31/1, [ssi_clk_divider]
  Switch1/1 -> Delay1/1, [ssi_encoder_bit_width_single_turn]
  Delay1/1 -> Switch1/3
  ssi_encoder_bit_width_single_turn_AXI/1 -> Delay2/1
  Delay2/1 -> Switch1/1
  ssi_data_in/1 -> Delay3/1
  Delay127/1 -> ssi_clk/1
  Delay3/1 -> [ssi_data_in]
  Switch6/1 -> [ssi_position_mech_single_turn_raw], position_raw_single_turn/1, Delay16/1, Delay15/1
  Delay4/1 -> RW_clk/1
  Delay7/1 -> RW_data/1
  Constant1/1 -> Delay4/1
  Constant3/1 -> Delay7/1
  Switch2/1 -> Delay8/1, [reciprocal_bit_width_single_turn]
  Delay9/1 -> Switch2/1
  Delay8/1 -> Switch2/3
  Delay10/1 -> position_mech_SI_single_turn/1
  Delay11/1 -> position_mech_SI_single_turn_AXI/1
  [ST_raw_with_offset_and_wrapped] -> Delay/1
  delay_first_clk_on_off_AXI/1 -> Delay6/1
  Delay6/1 -> Switch5/1
  Delay14/1 -> Switch5/3
  Switch5/1 -> [delay_first_clk_off_on], Delay14/1
  Delay15/1 -> Switch6/3
  Delay16/1 -> position_raw_single_turn_AXI/1
  Delay17/1 -> ssi_data_out_SH/1
  reciprocal_bit_width_single_turn_AXI/1 -> Delay9/1
  Product/1 -> Delay26/1
  [position_mech_si_with_offset_and_wrapped] -> Switch9/3
  position_to_speed_pll/1(speed_mech_SI) -> [speed_mech_SI]
  Switch23/1 -> Delay59/1, Delay18/1, Delay19/1
  Delay19/1 -> speed_mech_SI/1
  Delay18/1 -> speed_mech_SI_AXI/1
  Delay20/1 -> Switch3/3
  Delay21/1 -> Switch3/1
  Switch3/1 -> position_to_speed_pll/2(t_sample), Delay20/1
  Switch4/1 -> position_to_speed_pll/3(kp_pll), Delay22/1
  Delay23/1 -> Switch4/1
  Delay22/1 -> Switch4/3
  Switch7/1 -> position_to_speed_pll/4(ki_pll), Delay24/1
  Delay25/1 -> Switch7/1
  Delay24/1 -> Switch7/3
  t_sample_AXI/1 -> Delay21/1
  kp_pll_AXI/1 -> Delay23/1
  ki_pll_AXI/1 -> Delay25/1
  Delay/1 -> Product/1
  [reciprocal_bit_width_single_turn] -> Product/2
  Delay26/1 -> Product7/1
  Product7/1 -> [position_mech_si_with_offset_and_wrapped]
  Switch8/1 -> [debug_off_on], Delay27/1
  Delay28/1 -> Switch8/1
  Delay27/1 -> Switch8/3
  Switch9/1 -> position_to_speed_pll/1(position_mech_SI)
  Delay30/1 -> Switch10/1
  Delay29/1 -> Switch10/3
  Switch10/1 -> [position_mech_SI_debug], Delay29/1
  [debug_off_on] -> Switch9/2
  debug_off_on_AXI/1 -> Delay28/1
  position_mech_SI_debug_in_AXI/1 -> Delay30/1
  [position_mech_SI_debug] -> Switch9/1
  Constant4/1 -> Product1/2
  [speed_mech_SI] -> Product1/1
  Delay33/1 -> speed_mech_rpm/1
  Delay34/1 -> speed_mech_rpm_AXI/1
  Delay35/1 -> Switch11/3
  machine_polepairs_AXI/1 -> Delay36/1
  Delay36/1 -> Data Type Conversion/1
  Switch11/1 -> [machine_polepairs], Delay35/1
  Data Type Conversion/1 -> Switch11/1
  Detect Rise Positive1/1 -> [trigger_ssi_transaction], Switch18/2, Switch13/2, Switch31/2, Switch1/2, Switch15/2, Switch5/2, Switch20/2, Switch2/2, position_to_speed_pll/Trigger, Switch3/2, Switch4/2, Switch12/2, Switch11/2, Switch10/2, Switch8/2, Switch7/2, Switch14/2  "trigger_ssi"
  position_mech_offset_ticks_AXI/1 -> Delay38/1
  Switch12/1 -> [offset_ticks], Delay37/1
  Delay38/1 -> Switch12/1
  Delay37/1 -> Switch12/3
  [machine_polepairs] -> Product4/2
  [position_mech_si_with_offset_and_wrapped] -> Delay39/1
  Product4/1 -> Delay43/1
  Switch22/1 -> Delay11/1, Delay10/1, Delay58/1
  Delay39/1 -> Product4/1
  Delay42/1 -> position_el_SI_AXI/1
  Delay40/1 -> position_el_SI/1
  Delay43/1 -> wrap_2pi/1(input)
  Delay44/1 -> Switch13/3
  Switch13/1 -> Delay44/1, [ssi_encoder_bit_width_multi_turn]
  Delay45/1 -> Switch13/1
  ssi_encoder_bit_width_multi_turn_AXI/1 -> Delay45/1
  pos_is_binary_or_gray_AXI/1 -> Delay47/1
  Delay46/1 -> Switch14/3
  Delay47/1 -> Switch14/1
  Switch14/1 -> Delay46/1, [pos_is_binary_or_gray]
  Delay49/1 -> Switch15/1
  Switch15/1 -> Delay48/1, [ssi_encoder_number_of_status_bits]
  ssi_encoder_number_of_status_bits_AXI/1 -> Delay49/1
  Delay48/1 -> Switch15/3
  Switch16/1 -> Delay50/1, position_raw_multi_turn/1, [ssi_position_mech_multi_turn_raw], Delay51/1
  Delay51/1 -> position_raw_multi_turn_AXI/1
  Delay50/1 -> Switch16/3
  Constant/1 -> Product7/2
  OR/1 -> Switch17/1
  AND/1 -> S-R Flip-Flop1/1
  Constant5/1 -> Switch17/3
  Delay53/1 -> Switch18/1
  ssi_com_enable_AXI/1 -> Delay53/1
  Switch18/1 -> [ssi_com_enable], Delay52/1
  Delay52/1 -> Switch18/3
  [ssi_com_enable] -> AND/2, NOT1/1
  NOT/1 -> AND1/1, AND/1
  [ssi_clk_enb_out] -> NOT/1
  S-R Flip-Flop1/2 -> Terminator/1
  S-R Flip-Flop1/1 -> Switch17/2
  NOT1/1 -> Detect Rise Positive/1
  Detect Rise Positive/1 -> AND1/2
  Delay54/1 -> Switch19/3
  Switch19/1 -> status_raw/1, Delay55/1, Delay54/1
  Delay55/1 -> status_raw_AXI/1
  [ssi_data_out] -> Delay17/1
  [status_raw] -> Switch19/1
  AND1/1 -> S-R Flip-Flop1/2
  [speed_mech_SI] -> Product2/1
  Delay56/1 -> speed_el_SI/1
  [machine_polepairs] -> Product2/2
  Delay57/1 -> speed_el_SI_AXI/1
  Data Type Conversion1/1 -> slice_position_and_status/6(shift_val_st)
  [ssi_encoder_number_of_status_bits] -> Data Type Conversion1/1, Sum2/2, slice_position_and_status/4(bit_width_status)
  Sum2/1 -> slice_position_and_status/5(shift_val_mt)
  [ssi_encoder_bit_width_single_turn] -> Sum2/1, slice_position_and_status/3(bit_width_st)
  [pos_is_binary_or_gray] -> Gray_code_to_binary/2(pos_is_binary_or_gray)
  slice_position_and_status/1(pos_raw_st) -> Switch6/1  "pos_bin_st"
  slice_position_and_status/2(pos_raw_mt) -> Switch16/1  "pos_bin_mt"
  slice_position_and_status/3(raw_status) -> [status_raw]  "status_raw"
  [ssi_transaction_done] -> Delay129/1
  [ssi_clk_idle_levels] -> OR/2
  [trigger_ssi_transaction] -> ssi_communication/2(ssi_clk_reset)
  [ssi_encoder_bit_width_single_turn] -> ssi_communication/3(In3)
  [ssi_encoder_bit_width_multi_turn] -> ssi_communication/4(In4)
  [ssi_encoder_number_of_status_bits] -> ssi_communication/5(In5)
  [trigger_ssi_transaction] -> ssi_communication/7(trigger_ssi)
  ssi_communication/1(ssi_clk) -> [ssi_clk]
  ssi_communication/2(ssi_clk_enb_out) -> [ssi_clk_enb_out]
  ssi_communication/3(ssi_clk_idle_levels) -> [ssi_clk_idle_levels]
  ssi_communication/4(ssi_data_raw) -> [ssi_data_raw]
  ssi_communication/5(ssi_data_out) -> [ssi_data_out]
  ssi_communication/6(ssi_transaction_done) -> [ssi_transaction_done]
  [delay_first_clk_off_on] -> ssi_communication/6(delay_first_clk_on_off)
  [ssi_clk_divider] -> ssi_communication/1(ssi_clk_divider)
  [ssi_clk] -> OR/1
  [ssi_data_in] -> ssi_communication/8(ssi_data_in)
  Switch17/1 -> Delay127/1
  [ssi_transaction_done] -> Gray_code_to_binary/3(trigger)
  [ssi_data_raw] -> Gray_code_to_binary/1(ssi_data_raw)
  [ssi_encoder_bit_width_multi_turn] -> slice_position_and_status/2(bit_width_mt)
  [sampling_delay_clk_ticks] -> ssi_communication/9(sampling_delay_clk_ticks)
  Delay12/1 -> Switch20/1
  Delay5/1 -> Switch20/3
  sampling_delay_clk_ticks_AXI/1 -> Delay12/1
  Switch20/1 -> [sampling_delay_clk_ticks], Delay5/1
  Gray_code_to_binary/1(ssi_pos_binary) -> slice_position_and_status/1(data)
  Switch21/1 -> Delay13/1, position_multi_turn/1, Delay41/1
  Delay13/1 -> Switch21/3
  Delay41/1 -> position_multi_turn_AXI/1
  [trigger_ssi_transaction] -> Switch6/2, Switch16/2, Switch23/2, Switch24/2, Switch25/2, Switch26/2, Switch21/2, Switch22/2, Switch19/2
  [MT_raw_with_offset_and_wrapped] -> Switch21/1
  Delay58/1 -> Switch22/3
  [position_mech_si_with_offset_and_wrapped] -> Switch22/1
  [ssi_position_mech_multi_turn_raw] -> set_offset_to_raw_position_and_wrap/1(mt_raw)  "mt_raw"
  [ssi_encoder_bit_width_single_turn] -> set_offset_to_raw_position_and_wrap/2(n)  "n"
  [ssi_position_mech_single_turn_raw] -> set_offset_to_raw_position_and_wrap/3(st_raw)  "st_raw"
  [offset_ticks] -> set_offset_to_raw_position_and_wrap/4(In4)
  [ssi_encoder_bit_width_multi_turn] -> set_offset_to_raw_position_and_wrap/5(n1)  "n"
  set_offset_to_raw_position_and_wrap/1(st_raw_with_offset_and_wrapped) -> [ST_raw_with_offset_and_wrapped]
  set_offset_to_raw_position_and_wrap/2(mt_raw_with_offset_and_wrapped) -> [MT_raw_with_offset_and_wrapped]
  [speed_mech_SI] -> Switch23/1
  Delay59/1 -> Switch23/3
  Delay60/1 -> Switch24/3
  Switch24/1 -> Delay60/1, Delay56/1, Delay57/1
  Delay61/1 -> Switch25/3
  Switch25/1 -> Delay61/1, Delay34/1, Delay33/1
  Delay62/1 -> Switch26/3
  Switch26/1 -> Delay62/1, Delay42/1, Delay40/1
  wrap_2pi/1(output) -> Switch26/1
  Product1/1 -> Switch25/1
  Product2/1 -> Switch24/1

== system uz_ssi_interface_2025b/uz_ssi_interface/Gray_code_to_binary ==
  ssi_data_raw : Inport
  pos_is_binary_or_gray : Inport  Port=2
  trigger : Inport  Port=3
  Delay : Delay  DelayLength=1
  Delay2 : Delay  DelayLength=101
  Delay6 : Delay  DelayLength=1
  Switch : Switch  Criteria=u2 > Threshold  SaturateOnIntegerOverflow=off  InputSameDT=off
  gray_to_bin : Subsystem
  ssi_pos_binary : Outport
  wires:
  pos_is_binary_or_gray/1 -> Switch/2
  Switch/1 -> ssi_pos_binary/1
  ssi_data_raw/1 -> Delay2/1, Delay/1
  Delay/1 -> gray_to_bin/1(gray)
  Delay2/1 -> Switch/3
  Delay6/1 -> Switch/1
  trigger/1 -> gray_to_bin/2(enb)
  gray_to_bin/1(binary_out) -> Delay6/1
